simulink model "SF004B_AssiSumLim"  (R2013b)
settings: Solver=FixedStepDiscrete  StartTime=0.0  StopTime=1  FixedStep=.002  RelTol=1e-3
values from neighbouring files (symbols this model uses):
  AssiSumLimNtc0x0C4FailStep = DataDict.Calibration    [SF004B_AssiSumLim_DataDict.m]
  AssiSumLimNtc0x0C4PassStep = DataDict.Calibration    [SF004B_AssiSumLim_DataDict.m]
  AssiSumLimPullCmpLim = DataDict.Calibration    [SF004B_AssiSumLim_DataDict.m]
  CMDTHD_MOTNWTMTR_F32 = DataDict.Constant    [SF004B_AssiSumLim_DataDict.m]
  E_NOT_OK = DataDict.Constant    [AR200A_ArSuprt_DataDict.m]
  E_OK = DataDict.Constant    [AR200A_ArSuprt_DataDict.m]
  MOTTQZERO_MOTNWTMTR_F32 = DataDict.Constant    [SF004B_AssiSumLim_DataDict.m]
  VEHSPDTHD_KPH_F32 = DataDict.Constant    [SF004B_AssiSumLim_DataDict.m]
undefined symbols (not defined in the file or in its folder): NtcNr1, NtcSts1, SigQlfr1
libraries: simulink x11, NexteerUtilities x7, NxtrSign x1, NxtrAbslt x1
(part 1 of 3)
settings Model: Creator=gz9frc  LastModifiedBy=gz9frc
settings DataIOCC: LimitDataPoints=off  SaveFormat=Structure  ReturnWorkspaceOutputs=on
settings OptimizationCC: BlockReduction=off  InlineParams=on  ZeroExternalMemoryAtStartup=off  ZeroInternalMemoryAtStartup=off  OptimizeModelRefInitCode=on  LifeSpan=1
settings DebuggingCC: SignalInfNanChecking=error  SignalRangeChecking=warning  UnderspecifiedInitializationDetection=Simplified  SolverPrmCheckMsg=error  InheritedTsInSrcMsg=error  DiscreteInheritContinuousMsg=error  SingleTaskRateTransMsg=error  TasksWithSamePriorityMsg=error  SigSpecEnsureSampleTimeMsg=error  CheckMatrixSingularityMsg=error  IntegerOverflowMsg=error  ParameterUnderflowMsg=error  ParameterPrecisionLossMsg=error  ParameterTunabilityLossMsg=error  FixptConstUnderflowMsg=warning  FixptConstOverflowMsg=warning  VectorMatrixConversionMsg=error  SignalLabelMismatchMsg=error  UnconnectedInputMsg=error  UnconnectedOutputMsg=error  UnconnectedLineMsg=error  SFcnCompatibilityMsg=error  UniqueDataStoreMsg=warning  BusObjectLabelMismatch=error  RootOutportRequireBusObject=error  AssertControl=DisableAll  ModelReferenceIOMsg=error  ModelReferenceVersionMismatchMessage=warning  ModelReferenceIOMismatchMessage=error  ModelReferenceCSMismatchMessage=warning  ModelReferenceDataLoggingMessage=error  StateNameClashWarn=warning  StrictBusMsg=ErrorOnBusTreatedAsVector  NonBusSignalsTreatedAsBus=error  SFUnexpectedBacktrackingDiag=error  SFInvalidInputDataAccessInChartInitDiag=error  SFNoUnconditionalDefaultTransitionDiag=error  SFTransitionOutsideNaturalParentDiag=error  SFUnconditionalTransitionShadowingDiag=error  SFUndirectedBroadcastEventsDiag=error
settings ModelReferenceCC: ModelReferenceNumInstancesAllowed=Single
settings RTWCC: SystemTargetFile=autosar.tlc  GenCodeOnly=on  TemplateMakefile=ert_default_tmf  Description=AUTOSAR  GenerateReport=on  ProcessScript=autosar_make_rtw_hook  LaunchReport=on
settings CodeAppCC: GenerateComments=off  IgnoreCustomStorageClasses=off  CustomSymbolStrType=$N$R$M  CustomSymbolStrBlkIO=$N$M  SimulinkBlockComments=off
settings STFCustomTargetCC: ParMdlRefBuildCompliant=on  CompOptLevelCompliant=on  IncludeMdlTerminateFcn=off  CombineOutputUpdateFcns=on  SuppressErrorStatus=on  ERTFirstTimeCompliant=on  ERTCustomFileBanners=on  SupportNonFinite=off  SupportComplex=off  SupportContinuousTime=off  SupportNonInlinedSFcns=off  MATLABClassNameForMDSCustomization=Simulink.SoftwareTarget.ERTCustomization  AutosarCompliant=on  GRTInterface=off  SystemTargetFile=autosar.tlc
settings ERTTargetCC: CodeReplacementLibrary=ANSI_C  ConcurrentExecutionCompliant=off  IncludeMdlTerminateFcn=off  SuppressErrorStatus=on  SupportNonFinite=off  SupportComplex=off  ModelStepFunctionPrototypeControlCompliant=off  CPPClassGenCompliant=off  AutosarCompliant=on  InlinedParameterPlacement=NonHierarchical  ERTCustomFileTemplate=example_file_process.tlc  EnableUserReplacementTypes=on

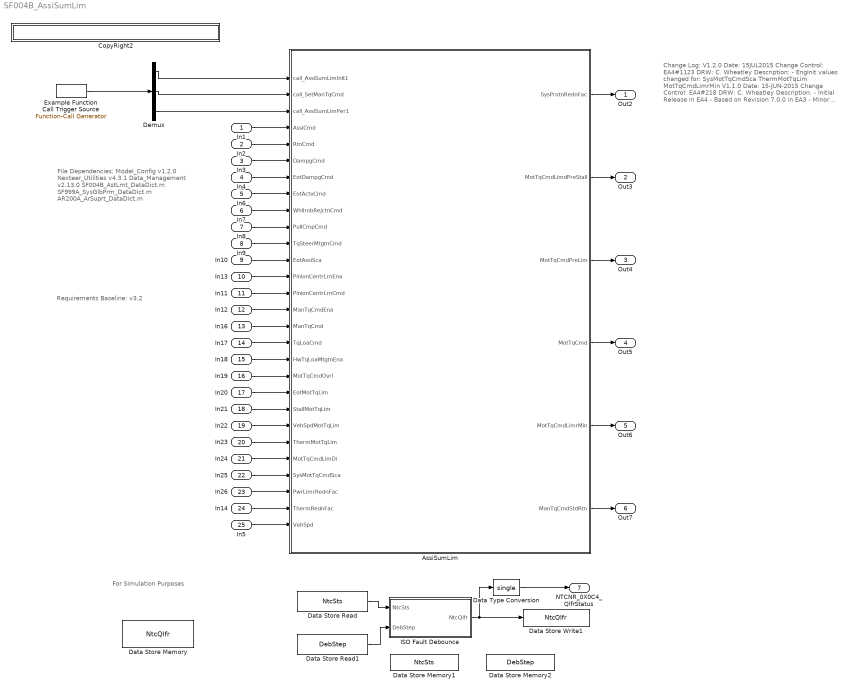
== system SF004B_AssiSumLim ==
  note: Requirements Baseline: v3.2
  note: Change Log:
      |
      | V1.2.0
      | Date: 15JUL2015
      | Change Control: EA4#1123
      | DRW: C. Wheatley
      | Description:
      | - EngInit values changed for:
      | 	SysMotTqCmdSca
      | 	ThermMotTqLim
      | 	MotTqCmdLimrMin
      |
      | V1.1.0
      | Date: 15-JUN-2015
      | Change Control: EA4#218
      | DRW: C. Wheatley
      | Description:
      | - Initial Release in EA4
      | - Based on Revision 7.0.0 in EA3
      | - Minor design change under EA4#746
  note: File Dependencies:
      |
      | Model_Config v1.2.0
      | Nexteer_Utilities v4.3.1
      | Data_Management v2.13.0
      | SF004B_AstLmt_DataDict.m
      | SF999A_SysGlbPrm_DataDict.m
      | AR200A_ArSuprt_DataDict.m
  note: For Simulation Purposes
  In1 : Inport
  In2 : Inport  Port=2
  In3 : Inport  Port=3
  In4 : Inport  Port=4
  In6 : Inport  Port=5
  In7 : Inport  Port=6
  In8 : Inport  Port=7
  In9 : Inport  Port=8
  In10 : Inport  Port=9
  In13 : Inport  Port=10
  In11 : Inport  Port=11
  In12 : Inport  Port=12
  In16 : Inport  Port=13
  In17 : Inport  Port=14
  In18 : Inport  Port=15
  In19 : Inport  Port=16
  In20 : Inport  Port=17
  In21 : Inport  Port=18
  In22 : Inport  Port=19
  In23 : Inport  Port=20
  In24 : Inport  Port=21
  In25 : Inport  Port=22
  In26 : Inport  Port=23
  In14 : Inport  Port=24
  In5 : Inport  Port=25
  AssiSumLim : Subsystem  RequirementInfo="{'linktype_rmi_doors' '00007fee (/E-STEER Core/SubSystem Specifications/Application Functions/SF004B Assist Summation and Limiting- Current)' '#SF004B_145' 'true' 'REQ:  SF004B_145' '' } %GIDa_c98ecf62_a109_47d6_a461_42c3ef856877"
  CopyRight2 : Subsystem  Description=|  mask(Copyright Information){none=on}
      | Copyright info block.                                               
      |                                                                     
      | Place copyright information at the top of every subsystem in design.
      mask prompts: none "No parameters"
      mask help: Place copyright information at the top of every subsystem in design.
      mask Display:
      | NxtrConf = 'Nexteer Confidential';
      | 
      | sys = bdroot; %handle for the current model ("system")
      | first = get_param(sys,'Created');
      | first = first(end-3:end);  %year is last four digits
      | 
      | last = get_param(sys,'LastModifiedDate');
      | if isempty(last)
      |     last = datestr(now,'yyyy');
      | else
      |     last = last(end-3:end);
      | end
      | 
      | if strcmp(first,last)
      |     fprintf('%s -- Copyright %s Nexteer',NxtrConf,first)
      | else
      |     fprintf('%s -- %s%s- %s Nexteer',NxtrConf,char(169),first,last)
      | end
  Data Store Memory : DataStoreMemory  DataStoreName=NtcQlfr  InitialValue=SigQlfr1.SIGQLFR_NORES  OutDataTypeStr=Enum: SigQlfr1
  Data Store Memory1 : DataStoreMemory  DataStoreName=NtcSts  InitialValue=NtcSts1.NTCSTS_PREPASSD
  Data Store Memory2 : DataStoreMemory  DataStoreName=DebStep
  Data Store Read : DataStoreRead  DataStoreName=NtcSts  SampleTime=0.002
  Data Store Read1 : DataStoreRead  DataStoreName=DebStep  SampleTime=0.002
  Data Store Write1 : DataStoreWrite  DataStoreName=NtcQlfr
  Data Type Conversion : DataTypeConversion  OutDataTypeStr=single
  Demux : Demux  Outputs=3
  Example Function Call Trigger Source : simulink/Ports & Subsystems/Function-Call Generator  RequirementInfo="{'linktype_rmi_doors' '00007fee (/E-STEER Core/SubSystem Specifications/Application Functions/SF004B Assist Summation and Limiting- Current)' '#SF004B_182' 'true' 'REQ:  SF004B_182' '' } %GIDa_fe8f626b_5d7f_45d0_99bb_2d66de232f0b"  sample_time=0.002  numberOfIterations=1
  ISO Fault Debounce : Subsystem
  Out2 : Outport
  Out3 : Outport  Port=2
  Out4 : Outport  Port=3
  Out5 : Outport  Port=4
  Out6 : Outport  Port=5
  Out7 : Outport  Port=6
  NTCNR_0X0C4_QlfrStatus : Outport  Port=7
  wires:
  Example Function Call Trigger Source/1 -> Demux/1
  AssiSumLim/3(MotTqCmdPreLim) -> Out4/1
  AssiSumLim/2(MotTqCmdLimdPreStall) -> Out3/1
  AssiSumLim/5(MotTqCmdLimrMin) -> Out6/1
  AssiSumLim/4(MotTqCmd) -> Out5/1
  AssiSumLim/1(SysProtnRednFac) -> Out2/1
  In4/1 -> AssiSumLim/7(EotDampgCmd)
  In26/1 -> AssiSumLim/26(PwrLimrRednFac)
  In24/1 -> AssiSumLim/24(MotTqCmdLimDi)
  In20/1 -> AssiSumLim/20(EotMotTqLim)
  In2/1 -> AssiSumLim/5(RtnCmd)
  In8/1 -> AssiSumLim/10(PullCmpCmd)
  In22/1 -> AssiSumLim/22(VehSpdMotTqLim)
  In6/1 -> AssiSumLim/8(EotActvCmd)
  In18/1 -> AssiSumLim/18(HwTqLoaMtgtnEna)
  In1/1 -> AssiSumLim/4(AssiCmd)
  In3/1 -> AssiSumLim/6(DampgCmd)
  In19/1 -> AssiSumLim/19(MotTqCmdOvrl)
  In17/1 -> AssiSumLim/17(TqLoaCmd)
  In23/1 -> AssiSumLim/23(ThermMotTqLim)
  In9/1 -> AssiSumLim/11(TqSteerMtgtnCmd)
  In21/1 -> AssiSumLim/21(StallMotTqLim)
  In11/1 -> AssiSumLim/14(PinionCentrLrnCmd)
  In25/1 -> AssiSumLim/25(SysMotTqCmdSca)
  In7/1 -> AssiSumLim/9(WhlImbRejctnCmd)
  In14/1 -> AssiSumLim/27(ThermRednFac)
  In5/1 -> AssiSumLim/28(VehSpd)
  In10/1 -> AssiSumLim/12(EotAssiSca)
  In13/1 -> AssiSumLim/13(PinionCentrLrnEna)
  Demux/3 -> AssiSumLim/3(call_AssiSumLimPer1)
  Demux/2 -> AssiSumLim/2(call_SetManTqCmd)
  Demux/1 -> AssiSumLim/1(call_AssiSumLimInit1)
  In16/1 -> AssiSumLim/16(ManTqCmd)
  In12/1 -> AssiSumLim/15(ManTqCmdEna)
  AssiSumLim/6(ManTqCmdStdRtn) -> Out7/1
  ISO Fault Debounce/1(NtcQlfr) -> Data Store Write1/1, Data Type Conversion/1
  Data Type Conversion/1 -> NTCNR_0X0C4_QlfrStatus/1
  Data Store Read/1 -> ISO Fault Debounce/1(NtcSts)
  Data Store Read1/1 -> ISO Fault Debounce/2(DebStep)

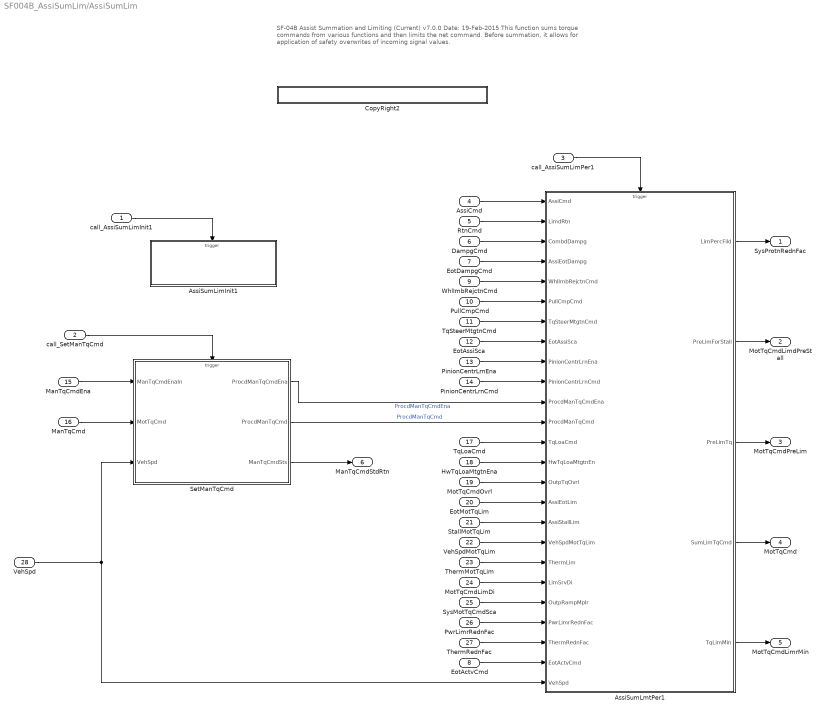
== system SF004B_AssiSumLim/AssiSumLim ==
  note: SF-04B Assist Summation and Limiting (Current)
      | v7.0.0 Date: 19-Feb-2015
      |
      | This function sums torque commands from various functions and then limits the net command.
      | Before summation, it allows for application of safety overwrites of incoming signal values.
  call_AssiSumLimInit1 : Inport
  call_SetManTqCmd : Inport  Port=2
  call_AssiSumLimPer1 : Inport  Port=3
  AssiCmd : Inport  RequirementInfo="{'linktype_rmi_doors' '00007fee (/E-STEER Core/SubSystem Specifications/Application Functions/SF004B Assist Summation and Limiting- Current)' '#SF004B_9' 'true' 'REQ:  SF004B_9' '' } %GIDa_bf460589_deb0_4830_baa9_957cfa45879d"  Port=4  PortDimensions=1
  RtnCmd : Inport  RequirementInfo="{'linktype_rmi_doors' '00007fee (/E-STEER Core/SubSystem Specifications/Application Functions/SF004B Assist Summation and Limiting- Current)' '#SF004B_33' 'true' 'REQ:  SF004B_33' '' } %GIDa_0c2bf6e9_dba7_44b0_b575_fa5eef1e919b"  Port=5  PortDimensions=1
  DampgCmd : Inport  RequirementInfo="{'linktype_rmi_doors' '00007fee (/E-STEER Core/SubSystem Specifications/Application Functions/SF004B Assist Summation and Limiting- Current)' '#SF004B_32' 'true' 'REQ:  SF004B_32' '' } %GIDa_eaacae62_eece_45d5_bf36_2cc76ecd952b"  Port=6  PortDimensions=1
  EotDampgCmd : Inport  RequirementInfo="{'linktype_rmi_doors' '00007fee (/E-STEER Core/SubSystem Specifications/Application Functions/SF004B Assist Summation and Limiting- Current)' '#SF004B_46' 'true' 'REQ:  SF004B_46' '' } %GIDa_a6be7234_a1fd_42a1_800c_3ec423f25189"  Port=7  PortDimensions=1
  EotActvCmd : Inport  RequirementInfo="{'linktype_rmi_doors' '00007fee (/E-STEER Core/SubSystem Specifications/Application Functions/SF004B Assist Summation and Limiting- Current)' '#SF004B_266' 'true' 'REQ:  SF004B_266' '' } %GIDa_53d43c83_1cf2_4e8a_981e_29e4c32f36c8"  Port=8  PortDimensions=1
  WhlImbRejctnCmd : Inport  RequirementInfo="{'linktype_rmi_doors' '00007fee (/E-STEER Core/SubSystem Specifications/Application Functions/SF004B Assist Summation and Limiting- Current)' '#SF004B_37' 'true' 'REQ:  SF004B_37' '' } %GIDa_c2e5f5ae_266a_4309_974e_4cf1a9d994f4"  Port=9  PortDimensions=1
  PullCmpCmd : Inport  RequirementInfo="{'linktype_rmi_doors' '00007fee (/E-STEER Core/SubSystem Specifications/Application Functions/SF004B Assist Summation and Limiting- Current)' '#SF004B_35' 'true' 'REQ:  SF004B_35' '' } %GIDa_c22ce321_48f2_40c4_abe6_caf9766843d3"  Port=10  PortDimensions=1
  TqSteerMtgtnCmd : Inport  RequirementInfo="{'linktype_rmi_doors' '00007fee (/E-STEER Core/SubSystem Specifications/Application Functions/SF004B Assist Summation and Limiting- Current)' '#SF004B_208' 'true' 'REQ:  SF004B_208' '' } %GIDa_25b38bed_c1c6_4303_9151_511a3f16d352"  Port=11
  EotAssiSca : Inport  RequirementInfo="{'linktype_rmi_doors' '00007fee (/E-STEER Core/SubSystem Specifications/Application Functions/SF004B Assist Summation and Limiting- Current)' '#SF004B_45' 'true' 'REQ:  SF004B_45' '' } %GIDa_60da6388_ce3f_4bb3_80ca_e73a484f5c2b"  Port=12  PortDimensions=1
  PinionCentrLrnEna : Inport  RequirementInfo="{'linktype_rmi_doors' '00007fee (/E-STEER Core/SubSystem Specifications/Application Functions/SF004B Assist Summation and Limiting- Current)' '#SF004B_267' 'true' 'REQ:  SF004B_267' '' } %GIDa_ba077a88_b1f9_4d8c_9c1a_953fa540ca74"  Port=13  PortDimensions=1
  PinionCentrLrnCmd : Inport  RequirementInfo="{'linktype_rmi_doors' '00007fee (/E-STEER Core/SubSystem Specifications/Application Functions/SF004B Assist Summation and Limiting- Current)' '#SF004B_269' 'true' 'REQ:  SF004B_269' '' } %GIDa_917054bb_73af_4ed2_8001_c85b7637104c"  Port=14  OutDataTypeStr=single  PortDimensions=1
  ManTqCmdEna : Inport  Port=15
  ManTqCmd : Inport  Port=16
  TqLoaCmd : Inport  RequirementInfo="{'linktype_rmi_doors' '00007fee (/E-STEER Core/SubSystem Specifications/Application Functions/SF004B Assist Summation and Limiting- Current)' '#SF004B_263' 'true' 'REQ:  SF004B_263' '' } %GIDa_87854b83_f54c_4612_b2c1_468ab820a899"  Port=17
  HwTqLoaMtgtnEna : Inport  RequirementInfo="{'linktype_rmi_doors' '00007fee (/E-STEER Core/SubSystem Specifications/Application Functions/SF004B Assist Summation and Limiting- Current)' '#SF004B_264' 'true' 'REQ:  SF004B_264' '' } %GIDa_f4d872e7_fa2f_4388_8a62_23bc86bbd1ee"  Port=18
  MotTqCmdOvrl : Inport  RequirementInfo="{'linktype_rmi_doors' '00007fee (/E-STEER Core/SubSystem Specifications/Application Functions/SF004B Assist Summation and Limiting- Current)' '#SF004B_34' 'true' 'REQ:  SF004B_34' '' } %GIDa_2478ccd5_9ac9_4740_8f5a_2a35a123e6f6"  Port=19  PortDimensions=1
  EotMotTqLim : Inport  RequirementInfo="{'linktype_rmi_doors' '00007fee (/E-STEER Core/SubSystem Specifications/Application Functions/SF004B Assist Summation and Limiting- Current)' '#SF004B_40' 'true' 'REQ:  SF004B_40' '' } %GIDa_f25ab945_aadc_4c90_aa23_83bff5c53583"  Port=20  PortDimensions=1
  StallMotTqLim : Inport  RequirementInfo="{'linktype_rmi_doors' '00007fee (/E-STEER Core/SubSystem Specifications/Application Functions/SF004B Assist Summation and Limiting- Current)' '#SF004B_39' 'true' 'REQ:  SF004B_39' '' } %GIDa_b8db5bfa_c139_4a26_8172_8da333f9ebcb"  Port=21  PortDimensions=1
  VehSpdMotTqLim : Inport  RequirementInfo="{'linktype_rmi_doors' '00007fee (/E-STEER Core/SubSystem Specifications/Application Functions/SF004B Assist Summation and Limiting- Current)' '#SF004B_38' 'true' 'REQ:  SF004B_38' '' } %GIDa_902cd062_b634_42fe_a170_6964bc658b1a"  Port=22  PortDimensions=1
  ThermMotTqLim : Inport  RequirementInfo="{'linktype_rmi_doors' '00007fee (/E-STEER Core/SubSystem Specifications/Application Functions/SF004B Assist Summation and Limiting- Current)' '#SF004B_41' 'true' 'REQ:  SF004B_41' '' } %GIDa_cc3ae51c_447a_4c5a_bdc3_a3c8d09ff335"  Port=23  PortDimensions=1
  MotTqCmdLimDi : Inport  RequirementInfo="{'linktype_rmi_doors' '00007fee (/E-STEER Core/SubSystem Specifications/Application Functions/SF004B Assist Summation and Limiting- Current)' '#SF004B_42' 'true' 'REQ:  SF004B_42' '' } %GIDa_df8fe6bc_32e8_4221_9558_4bad82c72033"  Port=24  PortDimensions=1
  SysMotTqCmdSca : Inport  RequirementInfo="{'linktype_rmi_doors' '00007fee (/E-STEER Core/SubSystem Specifications/Application Functions/SF004B Assist Summation and Limiting- Current)' '#SF004B_47' 'true' 'REQ:  SF004B_47' '' } %GIDa_f5b6de62_0cc3_467d_a951_ec2f549ed947"  Port=25  PortDimensions=1
  PwrLimrRednFac : Inport  RequirementInfo="{'linktype_rmi_doors' '00007fee (/E-STEER Core/SubSystem Specifications/Application Functions/SF004B Assist Summation and Limiting- Current)' '#SF004B_44' 'true' 'REQ:  SF004B_44' '' } %GIDa_4eba7841_fdd1_4f11_a699_a6f5b766d080"  Port=26  PortDimensions=1
  ThermRednFac : Inport  RequirementInfo="{'linktype_rmi_doors' '00007fee (/E-STEER Core/SubSystem Specifications/Application Functions/SF004B Assist Summation and Limiting- Current)' '#SF004B_43' 'true' 'REQ:  SF004B_43' '' } %GIDa_1c6e0acd_198a_4f88_bae4_afbebe03f547"  Port=27  PortDimensions=1
  VehSpd : Inport  RequirementInfo="{'linktype_rmi_doors' '00007fee (/E-STEER Core/SubSystem Specifications/Application Functions/SF004B Assist Summation and Limiting- Current)' '#SF004B_147' 'true' 'REQ:  SF004B_147' '' ; 'linktype_rmi_doors' '00007fee (/E-STEER Core/SubSystem Specifications/Application Functions/SF004B Assist Summation and Limiting- Current)' '#SF004B_283' 'true' 'REQ:  SF004B_283' '' } %GIDa_aade8552_3e00_42c2_86b7_eb68601364fe"  Port=28  PortDimensions=1
  AssiSumLimInit1 : Subsystem
  AssiSumLmtPer1 : Subsystem
  CopyRight2 : Subsystem  Description=|  mask(Copyright Information){none=on}
      | Copyright info block.                                               
      |                                                                     
      | Place copyright information at the top of every subsystem in design.
      mask prompts: none "No parameters"
      mask help: Place copyright information at the top of every subsystem in design.
      mask Display:
      | NxtrConf = 'Nexteer Confidential';
      | 
      | sys = bdroot; %handle for the current model ("system")
      | first = get_param(sys,'Created');
      | first = first(end-3:end);  %year is last four digits
      | 
      | last = get_param(sys,'LastModifiedDate');
      | if isempty(last)
      |     last = datestr(now,'yyyy');
      | else
      |     last = last(end-3:end);
      | end
      | 
      | if strcmp(first,last)
      |     fprintf('%s -- Copyright %s Nexteer',NxtrConf,first)
      | else
      |     fprintf('%s -- %s%s- %s Nexteer',NxtrConf,char(169),first,last)
      | end
  SetManTqCmd : Subsystem  RequirementInfo="{'linktype_rmi_doors' '00007fee (/E-STEER Core/SubSystem Specifications/Application Functions/SF004B Assist Summation and Limiting- Current)' '#SF004B_188' 'true' 'REQ:  SF004B_188' '' } %GIDa_6b8058f6_9489_4678_aa1c_db2b874903f9"
  SysProtnRednFac : Outport  RequirementInfo="{'linktype_rmi_doors' '00007fee (/E-STEER Core/SubSystem Specifications/Application Functions/SF004B Assist Summation and Limiting- Current)' '#SF004B_11' 'true' 'REQ:  SF004B_11' '' } %GIDa_7553187c_01cc_40b5_8c51_1ba61f1f9339"  PortDimensions=1
  MotTqCmdLimdPreStall : Outport  RequirementInfo="{'linktype_rmi_doors' '00007fee (/E-STEER Core/SubSystem Specifications/Application Functions/SF004B Assist Summation and Limiting- Current)' '#SF004B_53' 'true' 'REQ:  SF004B_53' '' } %GIDa_119b0193_ae9b_4bd5_baf4_512262ebe485"  Port=2  PortDimensions=1
  MotTqCmdPreLim : Outport  RequirementInfo="{'linktype_rmi_doors' '00007fee (/E-STEER Core/SubSystem Specifications/Application Functions/SF004B Assist Summation and Limiting- Current)' '#SF004B_52' 'true' 'REQ:  SF004B_52' '' } %GIDa_8ea21955_1860_43cf_a953_850b0c1ec6d7"  Port=3  PortDimensions=1
  MotTqCmd : Outport  RequirementInfo="{'linktype_rmi_doors' '00007fee (/E-STEER Core/SubSystem Specifications/Application Functions/SF004B Assist Summation and Limiting- Current)' '#SF004B_54' 'true' 'REQ:  SF004B_54' '' } %GIDa_1044b58a_41d3_48ab_88b4_80aeae3cd3c9"  Port=4  PortDimensions=1
  MotTqCmdLimrMin : Outport  RequirementInfo="{'linktype_rmi_doors' '00007fee (/E-STEER Core/SubSystem Specifications/Application Functions/SF004B Assist Summation and Limiting- Current)' '#SF004B_148' 'true' 'REQ:  SF004B_148' '' } %GIDa_6e0efbb3_baa3_4d1a_a57c_691bc3a103cb"  Port=5  PortDimensions=1
  ManTqCmdStdRtn : Outport  RequirementInfo="{'linktype_rmi_doors' '00007fee (/E-STEER Core/SubSystem Specifications/Application Functions/SF004B Assist Summation and Limiting- Current)' '#SF004B_148' 'true' 'REQ:  SF004B_148' '' } %GIDa_b5972cd0_2650_4f1d_9c34_049081f3f228"  Port=6  PortDimensions=1
  wires:
  AssiSumLmtPer1/5(TqLimMin) -> MotTqCmdLimrMin/1
  AssiSumLmtPer1/4(SumLimTqCmd) -> MotTqCmd/1
  AssiSumLmtPer1/3(PreLimTq) -> MotTqCmdPreLim/1
  AssiSumLmtPer1/2(PreLimForStall) -> MotTqCmdLimdPreStall/1
  AssiSumLmtPer1/1(LimPercFild) -> SysProtnRednFac/1
  call_AssiSumLimPer1/1 -> AssiSumLmtPer1/Trigger
  VehSpd/1 -> AssiSumLmtPer1/25(VehSpd), SetManTqCmd/3(VehSpd)
  AssiCmd/1 -> AssiSumLmtPer1/1(AssiCmd)
  RtnCmd/1 -> AssiSumLmtPer1/2(LimdRtn)
  DampgCmd/1 -> AssiSumLmtPer1/3(CombdDampg)
  EotDampgCmd/1 -> AssiSumLmtPer1/4(AssiEotDampg)
  WhlImbRejctnCmd/1 -> AssiSumLmtPer1/5(WhlImbRejctnCmd)
  PullCmpCmd/1 -> AssiSumLmtPer1/6(PullCmpCmd)
  TqSteerMtgtnCmd/1 -> AssiSumLmtPer1/7(TqSteerMtgtnCmd)
  EotAssiSca/1 -> AssiSumLmtPer1/8(EotAssiSca)
  TqLoaCmd/1 -> AssiSumLmtPer1/13(TqLoaCmd)
  HwTqLoaMtgtnEna/1 -> AssiSumLmtPer1/14(HwTqLoaMtgtnEn)
  MotTqCmdOvrl/1 -> AssiSumLmtPer1/15(OutpTqOvrl)
  EotMotTqLim/1 -> AssiSumLmtPer1/16(AssiEotLim)
  StallMotTqLim/1 -> AssiSumLmtPer1/17(AssiStallLim)
  VehSpdMotTqLim/1 -> AssiSumLmtPer1/18(VehSpdMotTqLim)
  ThermMotTqLim/1 -> AssiSumLmtPer1/19(ThermLim)
  MotTqCmdLimDi/1 -> AssiSumLmtPer1/20(LimSrvDi)
  SysMotTqCmdSca/1 -> AssiSumLmtPer1/21(OutpRampMplr)
  PwrLimrRednFac/1 -> AssiSumLmtPer1/22(PwrLimrRednFac)
  ThermRednFac/1 -> AssiSumLmtPer1/23(ThermRednFac)
  EotActvCmd/1 -> AssiSumLmtPer1/24(EotActvCmd)
  PinionCentrLrnEna/1 -> AssiSumLmtPer1/9(PinionCentrLrnEna)
  PinionCentrLrnCmd/1 -> AssiSumLmtPer1/10(PinionCentrLrnCmd)
  call_SetManTqCmd/1 -> SetManTqCmd/Trigger
  SetManTqCmd/3(ManTqCmdSts) -> ManTqCmdStdRtn/1
  call_AssiSumLimInit1/1 -> AssiSumLimInit1/Trigger
  ManTqCmdEna/1 -> SetManTqCmd/1(ManTqCmdEnaIn)
  ManTqCmd/1 -> SetManTqCmd/2(MotTqCmd)
  SetManTqCmd/1(ProcdManTqCmdEna) -> AssiSumLmtPer1/11(ProcdManTqCmdEna)  "ProcdManTqCmdEna"
  SetManTqCmd/2(ProcdManTqCmd) -> AssiSumLmtPer1/12(ProcdManTqCmd)  "ProcdManTqCmd"

== system SF004B_AssiSumLim/CopyRight2 ==

== system SF004B_AssiSumLim/ISO Fault Debounce ==
  note: Note:
      |
      | - "ISO Fault Debounce Design" Simulink block intent to use here for Simulation purpose only. Do not Code this block
  NtcSts : Inport
  DebStep : Inport  Port=2
  Constant : Constant  Value=false
  CopyRight2 : Subsystem  Description=|  mask(Copyright Information){none=on}
      | Copyright info block.                                               
      |                                                                     
      | Place copyright information at the top of every subsystem in design.
      mask prompts: none "No parameters"
      mask help: Place copyright information at the top of every subsystem in design.
      mask Display:
      | NxtrConf = 'Nexteer Confidential';
      | 
      | sys = bdroot; %handle for the current model ("system")
      | first = get_param(sys,'Created');
      | first = first(end-3:end);  %year is last four digits
      | 
      | last = get_param(sys,'LastModifiedDate');
      | if isempty(last)
      |     last = datestr(now,'yyyy');
      | else
      |     last = last(end-3:end);
      | end
      | 
      | if strcmp(first,last)
      |     fprintf('%s -- Copyright %s Nexteer',NxtrConf,first)
      | else
      |     fprintf('%s -- %s%s- %s Nexteer',NxtrConf,char(169),first,last)
      | end
  Data Type Conversion : DataTypeConversion
  DiagMgr : Subsystem  RequirementInfo="{'linktype_rmi_doors' '00007fee (/E-STEER Core/SubSystem Specifications/Application Functions/SF004B Assist Summation and Limiting- Current)' '#SF004B_271' 'true' 'REQ:  SF004B_271' '' ; 'linktype_rmi_doors' '00007fee (/E-STEER Core/SubSystem Specifications/Application Functions/SF004B Assist Summation and Limiting- Current)' '#SF004B_270' 'true' 'REQ:  SF004B_270' '' ; 'linktype_rmi_doors' '00007fee (/E-STEER Core/SubSystem Specifications/Application Functions/SF004B Assist Summation and Limiting- Current)' '#SF004B_272' 'true' 'REQ:  SF004B_272' '' ; 'linktype_rmi_doors' '00007fee (/E-STEER Core/SubSystem Specifications/Application Functions/SF004B Assist Summation and Limiting- Current)' '#SF004B_273' 'true' 'REQ:  SF004B_273' '' } %GIDa_c052514b_87e2_4362_ad4f_c7387e500b40"
  Ground : Ground
  Scope1 : Scope
  Scope2 : Scope
      settings: SaveName=ScopeData2
  Terminator : Terminator
  NtcQlfr : Outport
  wires:
  Ground/1 -> DiagMgr/3(SvcClr)
  DebStep/1 -> DiagMgr/2(DebStep), Scope2/1
  NtcSts/1 -> DiagMgr/1(NtcSts), Scope1/1
  Constant/1 -> DiagMgr/4(Recoverable)
  Data Type Conversion/1 -> NtcQlfr/1
  DiagMgr/1(Qualifier) -> Data Type Conversion/1
  DiagMgr/2(ErrAcc) -> Terminator/1

== system SF004B_AssiSumLim/AssiSumLim/AssiSumLimInit1 ==
  note: This component monitors Learn Pinion Center signals for safety violations, and sets a
      | Nexteer Trouble Code when a violation persists.
      |
      | This initialization runnable calls DiagMgr to set the NTC status to Pass.
  function : TriggerPort  TriggerType=function-call  PortDimensions=1
  Constant2 : Constant  Value=AssiSumLimNtc0x0C4PassStep
  Constant4 : Constant  Value=0
  CopyRight2 : Subsystem  Description=|  mask(Copyright Information){none=on}
      | Copyright info block.                                               
      |                                                                     
      | Place copyright information at the top of every subsystem in design.
      mask prompts: none "No parameters"
      mask help: Place copyright information at the top of every subsystem in design.
      mask Display:
      | NxtrConf = 'Nexteer Confidential';
      | 
      | sys = bdroot; %handle for the current model ("system")
      | first = get_param(sys,'Created');
      | first = first(end-3:end);  %year is last four digits
      | 
      | last = get_param(sys,'LastModifiedDate');
      | if isempty(last)
      |     last = datestr(now,'yyyy');
      | else
      |     last = last(end-3:end);
      | end
      | 
      | if strcmp(first,last)
      |     fprintf('%s -- Copyright %s Nexteer',NxtrConf,first)
      | else
      |     fprintf('%s -- %s%s- %s Nexteer',NxtrConf,char(169),first,last)
      | end
  Enumerated Constant1 : simulink/Sources/Enumerated Constant  OutDataTypeStr=Enum: NtcNr1  Value=NtcNr1.NTCNR_0X0C4  SampleTime=inf
  Enumerated Constant4 : simulink/Sources/Enumerated Constant  OutDataTypeStr=Enum: NtcSts1  Value=NtcSts1.NTCSTS_PASSD  SampleTime=inf
  SetNtcSts : Subsystem  mask(SetNTC){}
      mask help: SetNTC library block
  wires:
  Enumerated Constant1/1 -> SetNtcSts/1(NtcNr)
  Constant4/1 -> SetNtcSts/2(NtcStInfo)
  Enumerated Constant4/1 -> SetNtcSts/3(NtcSts)
  Constant2/1 -> SetNtcSts/4(DebStep)

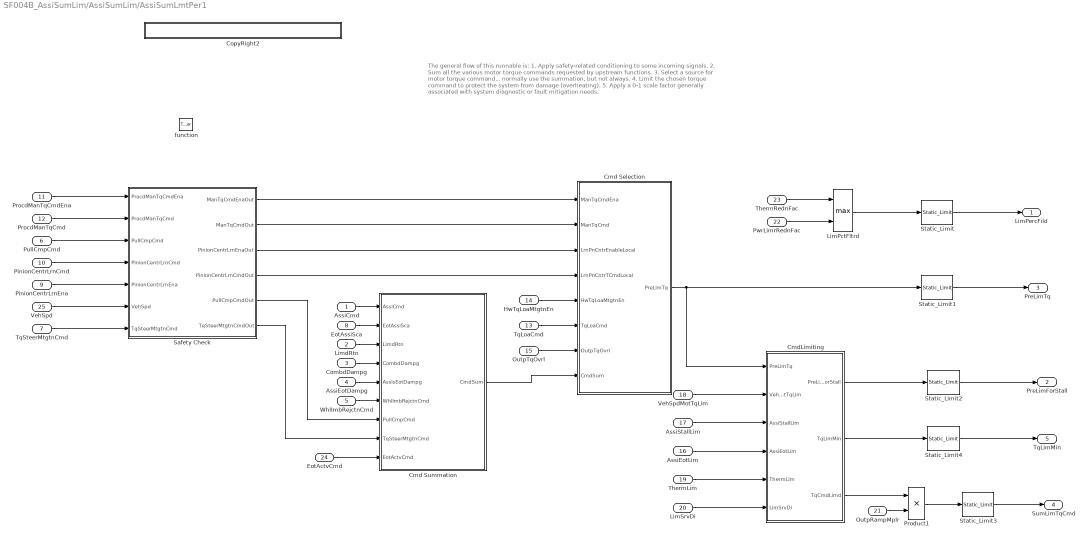
== system SF004B_AssiSumLim/AssiSumLim/AssiSumLmtPer1 ==
  note: The general flow of this runnable is:
      | 1.  Apply safety-related conditioning to some incoming signals.
      | 2.  Sum all the various motor torque commands requested by upstream functions.
      | 3.  Select a source for motor torque command... normally use the summation, but not always.
      | 4.  Limit the chosen torque command to protect the system from damage (overheating).
      | 5.  Apply a 0-1 scale factor generally associated with system diagnostic or fault mitigation needs.
  AssiCmd : Inport  PortDimensions=1
  LimdRtn : Inport  Port=2  PortDimensions=1
  CombdDampg : Inport  Port=3  PortDimensions=1
  AssiEotDampg : Inport  Port=4  PortDimensions=1
  WhlImbRejctnCmd : Inport  Port=5  PortDimensions=1
  PullCmpCmd : Inport  Port=6  PortDimensions=1
  TqSteerMtgtnCmd : Inport  RequirementInfo={} %GIDa_9ab500ab_7de2_465a_878f_aacb0693ce29  Port=7
  EotAssiSca : Inport  Port=8  PortDimensions=1
  PinionCentrLrnEna : Inport  Port=9  PortDimensions=1
  PinionCentrLrnCmd : Inport  Port=10  PortDimensions=1
  ProcdManTqCmdEna : Inport  Port=11  OutDataTypeStr=boolean  PortDimensions=1
  ProcdManTqCmd : Inport  Port=12  PortDimensions=1
  TqLoaCmd : Inport  Port=13  PortDimensions=1
  HwTqLoaMtgtnEn : Inport  Port=14  PortDimensions=1
  OutpTqOvrl : Inport  Port=15  PortDimensions=1
  AssiEotLim : Inport  Port=16  PortDimensions=1
  AssiStallLim : Inport  Port=17  PortDimensions=1
  VehSpdMotTqLim : Inport  Port=18  PortDimensions=1
  ThermLim : Inport  Port=19  PortDimensions=1
  LimSrvDi : Inport  Port=20  PortDimensions=1
  OutpRampMplr : Inport  RequirementInfo="{'linktype_rmi_doors' '00007fee (/E-STEER Core/SubSystem Specifications/Application Functions/SF004B Assist Summation and Limiting- Current)' '#SF004B_235' 'true' 'REQ:  SF004B_235' '' } %GIDa_1818b294_ff4f_4079_93d5_811a1ba3fd29"  Port=21  PortDimensions=1
  PwrLimrRednFac : Inport  RequirementInfo="{'linktype_rmi_doors' '00007fee (/E-STEER Core/SubSystem Specifications/Application Functions/SF004B Assist Summation and Limiting- Current)' '#SF004B_230' 'true' 'REQ:  SF004B_230' '' } %GIDa_cf155a5f_342c_45f9_9ae4_4c0f8d6d93ea"  Port=22  PortDimensions=1
  ThermRednFac : Inport  RequirementInfo="{'linktype_rmi_doors' '00007fee (/E-STEER Core/SubSystem Specifications/Application Functions/SF004B Assist Summation and Limiting- Current)' '#SF004B_230' 'true' 'REQ:  SF004B_230' '' } %GIDa_8ccdfb36_5ee5_4861_b8b5_3c0bf72e6fe3"  Port=23  PortDimensions=1
  EotActvCmd : Inport  RequirementInfo={} %GIDa_237a5011_7a86_4fee_b97d_0cb5cbc04e45  Port=24  PortDimensions=1
  VehSpd : Inport  Port=25  PortDimensions=1
  function : TriggerPort  TriggerType=function-call  PortDimensions=1
  Cmd Selection : Subsystem
  Cmd Summation : Subsystem
  CmdLimiting : Subsystem  Description=/*** Apply Gain and Limit ***/
  CopyRight2 : Subsystem  Description=|  mask(Copyright Information){none=on}
      | Copyright info block.                                               
      |                                                                     
      | Place copyright information at the top of every subsystem in design.
      mask prompts: none "No parameters"
      mask help: Place copyright information at the top of every subsystem in design.
      mask Display:
      | NxtrConf = 'Nexteer Confidential';
      | 
      | sys = bdroot; %handle for the current model ("system")
      | first = get_param(sys,'Created');
      | first = first(end-3:end);  %year is last four digits
      | 
      | last = get_param(sys,'LastModifiedDate');
      | if isempty(last)
      |     last = datestr(now,'yyyy');
      | else
      |     last = last(end-3:end);
      | end
      | 
      | if strcmp(first,last)
      |     fprintf('%s -- Copyright %s Nexteer',NxtrConf,first)
      | else
      |     fprintf('%s -- %s%s- %s Nexteer',NxtrConf,char(169),first,last)
      | end
  LimPctFltrd : MinMax  RequirementInfo="{'linktype_rmi_doors' '00007fee (/E-STEER Core/SubSystem Specifications/Application Functions/SF004B Assist Summation and Limiting- Current)' '#SF004B_230' 'true' 'REQ:  SF004B_230' '' } %GIDa_71492825_6196_4009_896f_01f3ecfaaeb5"  Function=max  Inputs=2
  Product1 : Product  RequirementInfo="{'linktype_rmi_doors' '00007fee (/E-STEER Core/SubSystem Specifications/Application Functions/SF004B Assist Summation and Limiting- Current)' '#SF004B_235' 'true' 'REQ:  SF004B_235' '' } %GIDa_f28742bc_8705_4125_be78_9f1828f9fc19"  RndMeth=Zero
  Safety Check : Subsystem
  Static_Limit : NexteerUtilities/Static_Limit  RequirementInfo="{'linktype_rmi_doors' '00007fee (/E-STEER Core/SubSystem Specifications/Application Functions/SF004B Assist Summation and Limiting- Current)' '#SF004B_204' 'true' 'REQ:  SF004B_204' '' } %GIDa_da8f0896_de7c_4e1c_91ff_ec02f9080ca3"  uprlim=LIMPERCCMPLHILIM_ULS_F32  lwrlim=LIMPERCCMPLLOLIM_ULS_F32
      settings: AttributesFormatString=|
      | Upper: %<uprlim>
      | Lower: %<lwrlim>
  Static_Limit1 : NexteerUtilities/Static_Limit  RequirementInfo="{'linktype_rmi_doors' '00007fee (/E-STEER Core/SubSystem Specifications/Application Functions/SF004B Assist Summation and Limiting- Current)' '#SF004B_204' 'true' 'REQ:  SF004B_204' '' } %GIDa_abb2abfb_33a1_4451_a1f5_2428b586a353"  uprlim=SYSGLBPRMMOTTQCMDHILIM_MOTNWTMTR_F32  lwrlim=SYSGLBPRMMOTTQCMDLOWRLIM_MOTNWTMTR_F32
      settings: AttributesFormatString=|
      | Upper: %<uprlim>
      | Lower: %<lwrlim>
  Static_Limit2 : NexteerUtilities/Static_Limit  RequirementInfo="{'linktype_rmi_doors' '00007fee (/E-STEER Core/SubSystem Specifications/Application Functions/SF004B Assist Summation and Limiting- Current)' '#SF004B_204' 'true' 'REQ:  SF004B_204' '' } %GIDa_12b89e81_1e49_4866_920a_fa19db2b8d00"  uprlim=SYSGLBPRMMOTTQCMDHILIM_MOTNWTMTR_F32  lwrlim=MOTTQZERO_MOTNWTMTR_F32
      settings: AttributesFormatString=|
      | Upper: %<uprlim>
      | Lower: %<lwrlim>
  Static_Limit3 : NexteerUtilities/Static_Limit  RequirementInfo="{'linktype_rmi_doors' '00007fee (/E-STEER Core/SubSystem Specifications/Application Functions/SF004B Assist Summation and Limiting- Current)' '#SF004B_204' 'true' 'REQ:  SF004B_204' '' } %GIDa_ade15596_b971_4b0e_893e_533054817dc3"  uprlim=SYSGLBPRMMOTTQCMDHILIM_MOTNWTMTR_F32  lwrlim=SYSGLBPRMMOTTQCMDLOWRLIM_MOTNWTMTR_F32
      settings: AttributesFormatString=|
      | Upper: %<uprlim>
      | Lower: %<lwrlim>
  Static_Limit4 : NexteerUtilities/Static_Limit  RequirementInfo="{'linktype_rmi_doors' '00007fee (/E-STEER Core/SubSystem Specifications/Application Functions/SF004B Assist Summation and Limiting- Current)' '#SF004B_204' 'true' 'REQ:  SF004B_204' '' } %GIDa_fdb98bc9_0173_435b_aa7a_92a1c0d327b6"  uprlim=SYSGLBPRMMOTTQCMDHILIM_MOTNWTMTR_F32  lwrlim=MOTTQZERO_MOTNWTMTR_F32
      settings: AttributesFormatString=|
      | Upper: %<uprlim>
      | Lower: %<lwrlim>
  LimPercFild : Outport  RequirementInfo={} %GIDa_f2122691_5fce_4e5e_81c4_e220de455558  PortDimensions=1
  PreLimForStall : Outport  RequirementInfo={} %GIDa_129bfd16_2a0e_48dc_a62a_9527e376d97b  Port=2  PortDimensions=1
  PreLimTq : Outport  RequirementInfo={} %GIDa_93433387_9ed3_46e5_8cb3_8b80bd3e7d12  Port=3  PortDimensions=1
  SumLimTqCmd : Outport  RequirementInfo={} %GIDa_18c69bbf_08af_4528_aba3_fd97eec39e1c  Port=4  PortDimensions=1
  TqLimMin : Outport  RequirementInfo={} %GIDa_f530c0fe_4151_421c_aa28_2884b5f891fa  Port=5  PortDimensions=1
  wires:
  CmdLimiting/2(TqLimMin) -> Static_Limit4/1
  AssiEotLim/1 -> CmdLimiting/4(AssiEotLim)
  ThermLim/1 -> CmdLimiting/5(ThermLim)
  VehSpdMotTqLim/1 -> CmdLimiting/2(VehSpdMotTqLim)
  AssiStallLim/1 -> CmdLimiting/3(AssiStallLim)
  LimSrvDi/1 -> CmdLimiting/6(LimSrvDi)
  Static_Limit1/1 -> PreLimTq/1
  Static_Limit2/1 -> PreLimForStall/1
  Static_Limit4/1 -> TqLimMin/1
  ThermRednFac/1 -> LimPctFltrd/1
  PwrLimrRednFac/1 -> LimPctFltrd/2
  LimPctFltrd/1 -> Static_Limit/1
  Static_Limit/1 -> LimPercFild/1
  Static_Limit3/1 -> SumLimTqCmd/1
  CmdLimiting/1(PreLimForStall) -> Static_Limit2/1
  Cmd Selection/1(PreLimTq) -> CmdLimiting/1(PreLimTq), Static_Limit1/1
  OutpRampMplr/1 -> Product1/2
  CmdLimiting/3(TqCmdLimd) -> Product1/1
  HwTqLoaMtgtnEn/1 -> Cmd Selection/5(HwTqLoaMtgtnEn)
  TqLoaCmd/1 -> Cmd Selection/6(TqLoaCmd)
  OutpTqOvrl/1 -> Cmd Selection/7(OutpTqOvrl)
  Product1/1 -> Static_Limit3/1
  Cmd Summation/1(CmdSum) -> Cmd Selection/8(CmdSum)
  AssiCmd/1 -> Cmd Summation/1(AssiCmd)
  AssiEotDampg/1 -> Cmd Summation/5(AssisEotDampg)
  WhlImbRejctnCmd/1 -> Cmd Summation/6(WhlImbRejctnCmd)
  TqSteerMtgtnCmd/1 -> Safety Check/7(TqSteerMtgtnCmd)
  EotAssiSca/1 -> Cmd Summation/2(EotAssiSca)
  PullCmpCmd/1 -> Safety Check/3(PullCmpCmd)
  LimdRtn/1 -> Cmd Summation/3(LimdRtn)
  CombdDampg/1 -> Cmd Summation/4(CombdDampg)
  EotActvCmd/1 -> Cmd Summation/9(EotActvCmd)
  Safety Check/5(PullCmpCmdOut) -> Cmd Summation/7(PullCmpCmd)
  VehSpd/1 -> Safety Check/6(VehSpd)
  Safety Check/6(TqSteerMtgtnCmdOut) -> Cmd Summation/8(TqSteerMtgtnCmd)
  ProcdManTqCmdEna/1 -> Safety Check/1(ProcdManTqCmdEna)
  ProcdManTqCmd/1 -> Safety Check/2(ProcdManTqCmd)
  PinionCentrLrnEna/1 -> Safety Check/5(PinionCentrLrnEna)
  PinionCentrLrnCmd/1 -> Safety Check/4(PinionCentrLrnCmd)
  Safety Check/1(ManTqCmdEnaOut) -> Cmd Selection/1(ManTqCmdEna)
  Safety Check/2(ManTqCmdOut) -> Cmd Selection/2(ManTqCmd)
  Safety Check/3(PinionCentrLrnEnaOut) -> Cmd Selection/3(LrnPnCntrEnableLocal)
  Safety Check/4(PinionCentrLrnCmdOut) -> Cmd Selection/4(LrnPnCntrTCmdLocal)

== system SF004B_AssiSumLim/AssiSumLim/CopyRight2 ==

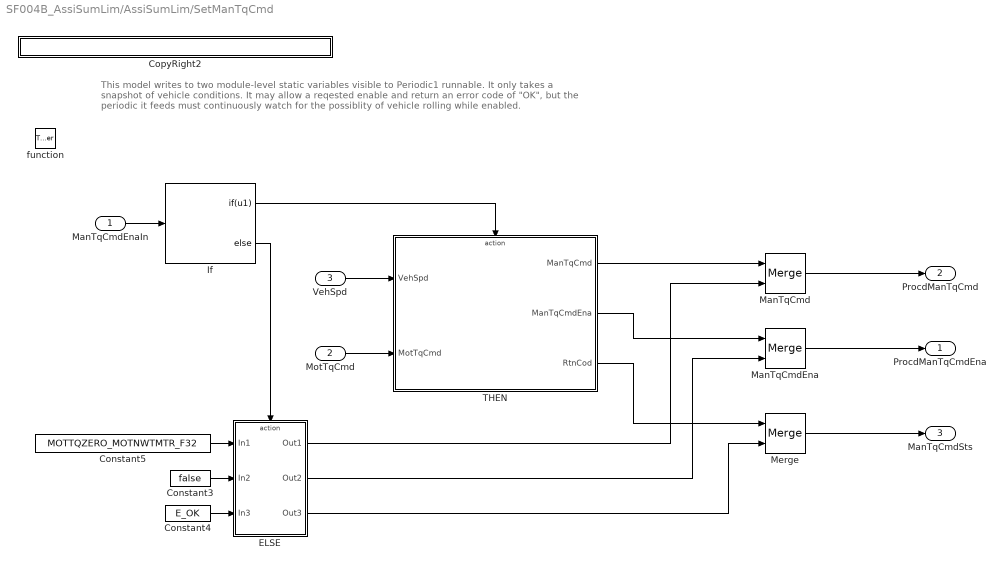
== system SF004B_AssiSumLim/AssiSumLim/SetManTqCmd ==
  note: This model writes to two module-level static variables visible to Periodic1 runnable.  It only takes a snapshot of vehicle conditions.  It may allow a reqested enable
      | and return an error code of "OK", but the periodic it feeds must continuously watch for the possiblity of vehicle rolling while enabled.
  ManTqCmdEnaIn : Inport  PortDimensions=1
  MotTqCmd : Inport  Port=2  PortDimensions=1
  VehSpd : Inport  Port=3  PortDimensions=1
  function : TriggerPort  TriggerType=function-call  PortDimensions=1
  Constant3 : Constant  RequirementInfo="{'linktype_rmi_doors' '00007fee (/E-STEER Core/SubSystem Specifications/Application Functions/SF004B Assist Summation and Limiting- Current)' '#SF004B_284' 'true' 'REQ:  SF004B_284' '' } %GIDa_246e7930_e475_402a_bdad_dd1be01de70c"  Value=false
  Constant4 : Constant  Value=E_OK
  Constant5 : Constant  RequirementInfo="{'linktype_rmi_doors' '00007fee (/E-STEER Core/SubSystem Specifications/Application Functions/SF004B Assist Summation and Limiting- Current)' '#SF004B_284' 'true' 'REQ:  SF004B_284' '' } %GIDa_0892c191_fb5f_47cd_b4da_28c04b362257"  Value=MOTTQZERO_MOTNWTMTR_F32
  CopyRight2 : Subsystem  Description=|  mask(Copyright Information){none=on}
      | Copyright info block.                                               
      |                                                                     
      | Place copyright information at the top of every subsystem in design.
      mask prompts: none "No parameters"
      mask help: Place copyright information at the top of every subsystem in design.
      mask Display:
      | NxtrConf = 'Nexteer Confidential';
      | 
      | sys = bdroot; %handle for the current model ("system")
      | first = get_param(sys,'Created');
      | first = first(end-3:end);  %year is last four digits
      | 
      | last = get_param(sys,'LastModifiedDate');
      | if isempty(last)
      |     last = datestr(now,'yyyy');
      | else
      |     last = last(end-3:end);
      | end
      | 
      | if strcmp(first,last)
      |     fprintf('%s -- Copyright %s Nexteer',NxtrConf,first)
      | else
      |     fprintf('%s -- %s%s- %s Nexteer',NxtrConf,char(169),first,last)
      | end
  ELSE : Subsystem  RequirementInfo="{'linktype_rmi_doors' '00007fee (/E-STEER Core/SubSystem Specifications/Application Functions/SF004B Assist Summation and Limiting- Current)' '#SF004B_284' 'true' 'REQ:  SF004B_284' '' } %GIDa_6bd0155f_980a_4aad_a811_84a5ccc9badc"  TreatAsAtomicUnit=on
      settings: RTWSystemCode=Inline
  If : If  RequirementInfo="{'linktype_rmi_doors' '00007fee (/E-STEER Core/SubSystem Specifications/Application Functions/SF004B Assist Summation and Limiting- Current)' '#SF004B_284' 'true' 'REQ:  SF004B_284' '' ; 'linktype_rmi_doors' '00007fee (/E-STEER Core/SubSystem Specifications/Application Functions/SF004B Assist Summation and Limiting- Current)' '#SF004B_285' 'true' 'REQ:  SF004B_285' '' ; 'linktype_rmi_doors' '00007fee (/E-STEER Core/SubSystem Specifications/Application Functions/SF004B Assist Summation and Limiting- Current)' '#SF004B_286' 'true' 'REQ:  SF004B_286' '' } %GIDa_76959808_7222_4e91_b5be_e00bbca0187f"  IfExpression=u1
  ManTqCmd : Merge
  ManTqCmdEna : Merge
  Merge : Merge
  THEN : Subsystem  RequirementInfo="{'linktype_rmi_doors' '00007fee (/E-STEER Core/SubSystem Specifications/Application Functions/SF004B Assist Summation and Limiting- Current)' '#SF004B_285' 'true' 'REQ:  SF004B_285' '' ; 'linktype_rmi_doors' '00007fee (/E-STEER Core/SubSystem Specifications/Application Functions/SF004B Assist Summation and Limiting- Current)' '#SF004B_286' 'true' 'REQ:  SF004B_286' '' } %GIDa_2fb8668e_6be1_4ac8_9f6e_6c48479f05c2"  TreatAsAtomicUnit=on
      settings: RTWSystemCode=Inline
  ProcdManTqCmdEna : Outport
  ProcdManTqCmd : Outport  Port=2
  ManTqCmdSts : Outport  RequirementInfo={} %GIDa_7e6f8e1d_b1f7_4fb4_abd3_4fdb315f2f2e  Port=3  PortDimensions=1
  wires:
  ManTqCmdEnaIn/1 -> If/1
  If/1 -> THEN/Action
  VehSpd/1 -> THEN/1(VehSpd)
  MotTqCmd/1 -> THEN/2(MotTqCmd)
  Constant5/1 -> ELSE/1(In1)
  Constant3/1 -> ELSE/2(In2)
  If/2 -> ELSE/Action
  Constant4/1 -> ELSE/3(In3)
  THEN/1(ManTqCmd) -> ManTqCmd/1
  ELSE/1(Out1) -> ManTqCmd/2
  THEN/2(ManTqCmdEna) -> ManTqCmdEna/1
  ELSE/2(Out2) -> ManTqCmdEna/2
  THEN/3(RtnCod) -> Merge/1
  ELSE/3(Out3) -> Merge/2
  ManTqCmd/1 -> ProcdManTqCmd/1
  ManTqCmdEna/1 -> ProcdManTqCmdEna/1
  Merge/1 -> ManTqCmdSts/1

== system SF004B_AssiSumLim/ISO Fault Debounce/CopyRight2 ==

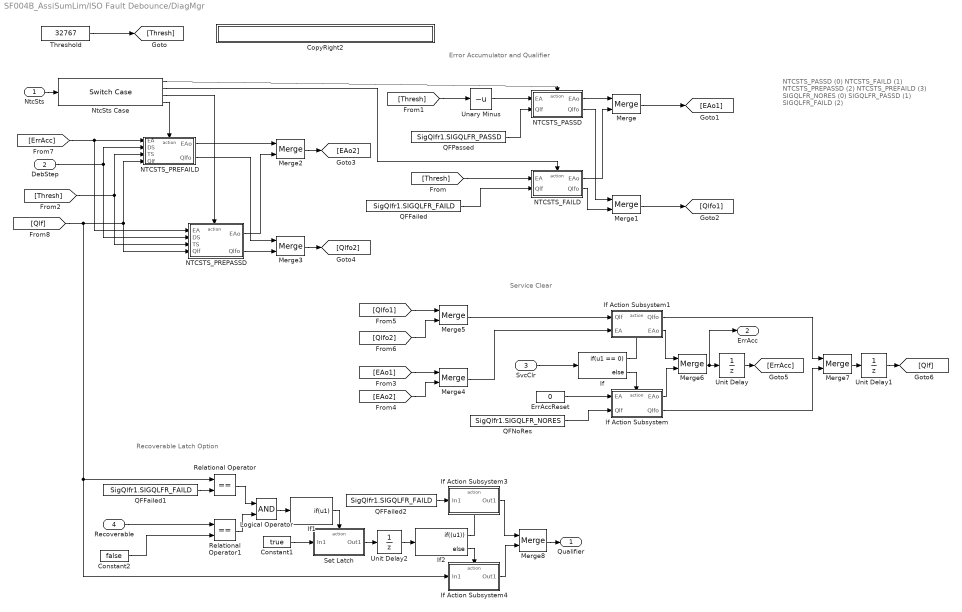
== system SF004B_AssiSumLim/ISO Fault Debounce/DiagMgr ==
  note: NTCSTS_PASSD         (0)
      | NTCSTS_FAILD           (1)
      | NTCSTS_PREPASSD  (2)
      | NTCSTS_PREFAILD    (3)
      |
      | SIGQLFR_NORES       (0)
      | SIGQLFR_PASSD        (1)
      | SIGQLFR_FAILD          (2)
  note: Error Accumulator and Qualifier
  note: Service Clear
  note: Recoverable Latch Option
  NtcSts : Inport
  DebStep : Inport  Port=2
  SvcClr : Inport  Port=3
  Recoverable : Inport  Port=4
  Constant1 : Constant  Value=true  OutDataTypeStr=boolean
  Constant2 : Constant  Value=false  OutDataTypeStr=boolean
  CopyRight2 : Subsystem  Description=|  mask(Copyright Information){none=on}
      | Copyright info block.                                               
      |                                                                     
      | Place copyright information at the top of every subsystem in design.
      mask prompts: none "No parameters"
      mask help: Place copyright information at the top of every subsystem in design.
      mask Display:
      | NxtrConf = 'Nexteer Confidential';
      | 
      | sys = bdroot; %handle for the current model ("system")
      | first = get_param(sys,'Created');
      | first = first(end-3:end);  %year is last four digits
      | 
      | last = get_param(sys,'LastModifiedDate');
      | if isempty(last)
      |     last = datestr(now,'yyyy');
      | else
      |     last = last(end-3:end);
      | end
      | 
      | if strcmp(first,last)
      |     fprintf('%s -- Copyright %s Nexteer',NxtrConf,first)
      | else
      |     fprintf('%s -- %s%s- %s Nexteer',NxtrConf,char(169),first,last)
      | end
  ErrAccReset : Constant  Value=0
  If : If  IfExpression=u1 == 0
  If Action Subsystem : Subsystem  TreatAsAtomicUnit=on
  If Action Subsystem1 : Subsystem  TreatAsAtomicUnit=on
  If Action Subsystem3 : Subsystem  TreatAsAtomicUnit=on
  If Action Subsystem4 : Subsystem  TreatAsAtomicUnit=on
  If1 : If  IfExpression=u1  ShowElse=off
  If2 : If  IfExpression=(u1)
  Logical Operator : Logic  AllPortsSameDT=off  OutDataTypeStr=boolean
  Merge{,1..8} (9 alike) : Merge
  NTCSTS_FAILD : Subsystem  TreatAsAtomicUnit=on
  NTCSTS_PASSD : Subsystem  TreatAsAtomicUnit=on
  NTCSTS_PREFAILD : Subsystem  TreatAsAtomicUnit=on
  NTCSTS_PREPASSD : Subsystem  TreatAsAtomicUnit=on
  NtcSts Case : SwitchCase  CaseConditions={NtcSts1.NTCSTS_PASSD,NtcSts1.NTCSTS_FAILD,NtcSts1.NTCSTS_PREPASSD,NtcSts1.NTCSTS_PREFAILD}  ShowDefaultCase=off
  QFFailed : Constant  Value=SigQlfr1.SIGQLFR_FAILD  OutDataTypeStr=Enum: SigQlfr1
  QFFailed1 : Constant  Value=SigQlfr1.SIGQLFR_FAILD  OutDataTypeStr=Enum: SigQlfr1
  QFFailed2 : Constant  Value=SigQlfr1.SIGQLFR_FAILD  OutDataTypeStr=Enum: SigQlfr1
  QFNoRes : Constant  Value=SigQlfr1.SIGQLFR_NORES  OutDataTypeStr=Enum: SigQlfr1
  QFPassed : Constant  Value=SigQlfr1.SIGQLFR_PASSD  OutDataTypeStr=Enum: SigQlfr1
  Relational Operator : RelationalOperator  Operator===  OutDataTypeStr=boolean
      settings: AttributesFormatString=Qualifier Failed
  Relational Operator1 : RelationalOperator  Operator===  OutDataTypeStr=boolean
      settings: AttributesFormatString=Recoverable False
  Set Latch : Subsystem  TreatAsAtomicUnit=on
  Threshold : Constant  Value=32767
  Unary Minus : UnaryMinus
  Unit Delay : UnitDelay  SampleTime=-1
  Unit Delay1 : UnitDelay  InitialCondition=SigQlfr1.SIGQLFR_NORES  SampleTime=-1  StateName=SigQlfr1
  Unit Delay2 : UnitDelay  SampleTime=-1
  Qualifier : Outport
  ErrAcc : Outport  Port=2
  wires:
  DebStep/1 -> NTCSTS_PREPASSD/2(DS), NTCSTS_PREFAILD/2(DS)
  NtcSts Case/3 -> NTCSTS_PREPASSD/Action
  If/2 -> If Action Subsystem/Action
  QFPassed/1 -> NTCSTS_PASSD/2(Qlf)
  If2/1 -> If Action Subsystem3/Action
  If2/2 -> If Action Subsystem4/Action
  [Thresh] -> NTCSTS_FAILD/1(EA)
  QFFailed/1 -> NTCSTS_FAILD/2(Qlf)
  If Action Subsystem4/1(Out1) -> Merge8/2
  Merge8/1 -> Qualifier/1
  QFFailed2/1 -> If Action Subsystem3/1(In1)
  Unit Delay2/1 -> If2/1
  NtcSts Case/1 -> NTCSTS_PASSD/Action
  NtcSts Case/4 -> NTCSTS_PREFAILD/Action
  SvcClr/1 -> If/1
  NtcSts Case/2 -> NTCSTS_FAILD/Action
  [Thresh] -> Unary Minus/1
  [Thresh] -> NTCSTS_PREPASSD/3(TS), NTCSTS_PREFAILD/3(TS)
  NTCSTS_PREFAILD/2(Qlfo) -> Merge3/1
  [ErrAcc] -> NTCSTS_PREPASSD/1(EA), NTCSTS_PREFAILD/1(EA)
  NTCSTS_PREPASSD/1(EAo) -> Merge2/2
  NTCSTS_FAILD/1(EAo) -> Merge/2
  NTCSTS_FAILD/2(Qlfo) -> Merge1/2
  If Action Subsystem3/1(Out1) -> Merge8/1
  [Qlfo1] -> Merge5/1
  NTCSTS_PREPASSD/2(Qlfo) -> Merge3/2
  NTCSTS_PREFAILD/1(EAo) -> Merge2/1
  [Qlfo2] -> Merge5/2
  [EAo1] -> Merge4/1
  [Qlf] -> Relational Operator/1, If Action Subsystem4/1(In1), NTCSTS_PREFAILD/4(Qlf), NTCSTS_PREPASSD/4(Qlf)
  [EAo2] -> Merge4/2
  Merge/1 -> [EAo1]
  ErrAccReset/1 -> If Action Subsystem/1(EA)
  QFNoRes/1 -> If Action Subsystem/2(Qlf)
  Merge6/1 -> ErrAcc/1, Unit Delay/1
  If Action Subsystem1/2(EAo) -> Merge6/1
  Merge4/1 -> If Action Subsystem1/2(EA)
  If/1 -> If Action Subsystem1/Action
  If Action Subsystem1/1(Qlfo) -> Merge7/1
  NTCSTS_PASSD/2(Qlfo) -> Merge1/1
  Threshold/1 -> [Thresh]
  If Action Subsystem/1(EAo) -> Merge6/2
  NTCSTS_PASSD/1(EAo) -> Merge/1
  If Action Subsystem/2(Qlfo) -> Merge7/2
  Merge1/1 -> [Qlfo1]
  Merge2/1 -> [EAo2]
  Merge3/1 -> [Qlfo2]
  Merge5/1 -> If Action Subsystem1/1(Qlf)
  NtcSts/1 -> NtcSts Case/1
  Unit Delay/1 -> [ErrAcc]
  Unit Delay1/1 -> [Qlf]
  Merge7/1 -> Unit Delay1/1
  Relational Operator/1 -> Logical Operator/1
  Relational Operator1/1 -> Logical Operator/2
  Constant2/1 -> Relational Operator1/2
  Logical Operator/1 -> If1/1
  If1/1 -> Set Latch/Action
  Constant1/1 -> Set Latch/1(In1)
  QFFailed1/1 -> Relational Operator/2
  Set Latch/1(Out1) -> Unit Delay2/1
  Recoverable/1 -> Relational Operator1/1
  Unary Minus/1 -> NTCSTS_PASSD/1(EA)

== system SF004B_AssiSumLim/AssiSumLim/AssiSumLimInit1/CopyRight2 ==

== system SF004B_AssiSumLim/AssiSumLim/AssiSumLimInit1/SetNtcSts ==
  NtcNr : Inport
  NtcStInfo : Inport  Port=2
  NtcSts : Inport  Port=3
  DebStep : Inport  Port=4
  Data Store Write1 : DataStoreWrite  DataStoreName=DebStep
  Data Store Write2 : DataStoreWrite  DataStoreName=NtcSts
  Terminator : Terminator
  Terminator1 : Terminator
  wires:
  NtcStInfo/1 -> Terminator1/1
  DebStep/1 -> Data Store Write1/1
  NtcSts/1 -> Data Store Write2/1
  NtcNr/1 -> Terminator/1
